simulink model "fangzhen"  (R2018a)
settings: Solver=FixedStepAuto  StartTime=0.0  StopTime=120  FixedStep=0.01  RelTol=1e-3
libraries: simulink x6
(part 2 of 2)

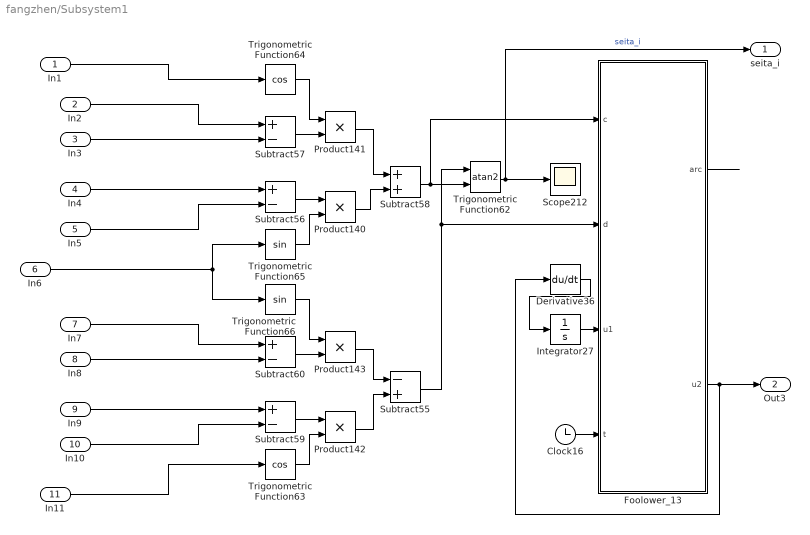
== system fangzhen/Subsystem1 ==
  In1 : Inport
  In2 : Inport  Port=2
  In3 : Inport  Port=3
  In4 : Inport  Port=4
  In5 : Inport  Port=5
  In6 : Inport  Port=6
  In7 : Inport  Port=7
  In8 : Inport  Port=8
  In9 : Inport  Port=9
  In10 : Inport  Port=10
  In11 : Inport  Port=11
  Clock16 : Clock
  Derivative36 : Derivative
  Foolower_13 : MATLAB Function  TreatAsAtomicUnit=on
  Integrator27 : Integrator
  Product{140..143} (4 alike) : Product
  Scope212 : Scope
  Subtract55 : Sum  Inputs=-+
  Subtract{56..57,59..60} (4 alike) : Sum  Inputs=+-
  Subtract58 : Sum
  Trigonometric Function62 : Trigonometry  Operator=atan2
  Trigonometric Function63 : Trigonometry  Operator=cos
  Trigonometric Function64 : Trigonometry  Operator=cos
  Trigonometric Function65 : Trigonometry
  Trigonometric Function66 : Trigonometry
  seita_i : Outport
  Out3 : Outport  Port=2
  wires:
  Foolower_13/2(u2) -> Out3/1, Derivative36/1
  Trigonometric Function64/1 -> Product141/1
  In6/1 -> Trigonometric Function66/1, Trigonometric Function65/1
  Trigonometric Function66/1 -> Product143/1
  Subtract58/1 -> Foolower_13/1(c), Trigonometric Function62/2
  In3/1 -> Subtract57/2
  Product142/1 -> Subtract55/2
  Subtract55/1 -> Trigonometric Function62/1, Foolower_13/2(d)
  Product143/1 -> Subtract55/1
  In10/1 -> Subtract59/2
  Subtract60/1 -> Product143/2
  Derivative36/1 -> Integrator27/1
  In9/1 -> Subtract59/1
  Trigonometric Function63/1 -> Product142/2
  Trigonometric Function62/1 -> seita_i/1, Scope212/1  "seita_i"
  Clock16/1 -> Foolower_13/4(t)
  In1/1 -> Trigonometric Function64/1
  Subtract56/1 -> Product140/1
  Integrator27/1 -> Foolower_13/3(u1)
  In5/1 -> Subtract56/2
  Subtract59/1 -> Product142/1
  Product141/1 -> Subtract58/1
  Foolower_13/1(arc) -> ?
  Product140/1 -> Subtract58/2
  In2/1 -> Subtract57/1
  Trigonometric Function65/1 -> Product140/2
  Subtract57/1 -> Product141/2
  In11/1 -> Trigonometric Function63/1
  In7/1 -> Subtract60/1
  In8/1 -> Subtract60/2
  In4/1 -> Subtract56/1

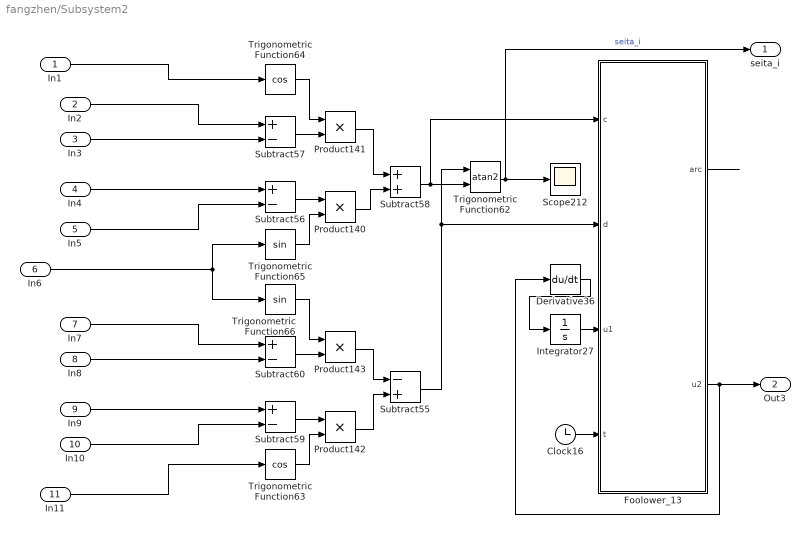
== system fangzhen/Subsystem2 ==
  In1 : Inport
  In2 : Inport  Port=2
  In3 : Inport  Port=3
  In4 : Inport  Port=4
  In5 : Inport  Port=5
  In6 : Inport  Port=6
  In7 : Inport  Port=7
  In8 : Inport  Port=8
  In9 : Inport  Port=9
  In10 : Inport  Port=10
  In11 : Inport  Port=11
  Clock16 : Clock
  Derivative36 : Derivative
  Foolower_13 : MATLAB Function  TreatAsAtomicUnit=on
  Integrator27 : Integrator
  Product{140..143} (4 alike) : Product
  Scope212 : Scope
  Subtract55 : Sum  Inputs=-+
  Subtract{56..57,59..60} (4 alike) : Sum  Inputs=+-
  Subtract58 : Sum
  Trigonometric Function62 : Trigonometry  Operator=atan2
  Trigonometric Function63 : Trigonometry  Operator=cos
  Trigonometric Function64 : Trigonometry  Operator=cos
  Trigonometric Function65 : Trigonometry
  Trigonometric Function66 : Trigonometry
  seita_i : Outport
  Out3 : Outport  Port=2
  wires:
  Foolower_13/2(u2) -> Out3/1, Derivative36/1
  Trigonometric Function64/1 -> Product141/1
  In6/1 -> Trigonometric Function66/1, Trigonometric Function65/1
  Trigonometric Function66/1 -> Product143/1
  Subtract58/1 -> Foolower_13/1(c), Trigonometric Function62/2
  In3/1 -> Subtract57/2
  Product142/1 -> Subtract55/2
  Subtract55/1 -> Trigonometric Function62/1, Foolower_13/2(d)
  Product143/1 -> Subtract55/1
  In10/1 -> Subtract59/2
  Subtract60/1 -> Product143/2
  Derivative36/1 -> Integrator27/1
  In9/1 -> Subtract59/1
  Trigonometric Function63/1 -> Product142/2
  Trigonometric Function62/1 -> seita_i/1, Scope212/1  "seita_i"
  Clock16/1 -> Foolower_13/4(t)
  In1/1 -> Trigonometric Function64/1
  Subtract56/1 -> Product140/1
  Integrator27/1 -> Foolower_13/3(u1)
  In5/1 -> Subtract56/2
  Subtract59/1 -> Product142/1
  Product141/1 -> Subtract58/1
  Foolower_13/1(arc) -> ?
  Product140/1 -> Subtract58/2
  In2/1 -> Subtract57/1
  Trigonometric Function65/1 -> Product140/2
  Subtract57/1 -> Product141/2
  In11/1 -> Trigonometric Function63/1
  In7/1 -> Subtract60/1
  In8/1 -> Subtract60/2
  In4/1 -> Subtract56/1

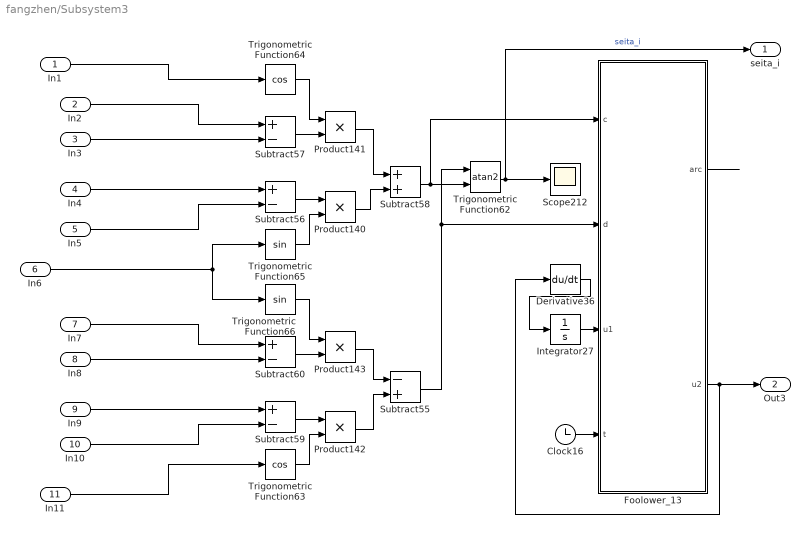
== system fangzhen/Subsystem3 ==
  In1 : Inport
  In2 : Inport  Port=2
  In3 : Inport  Port=3
  In4 : Inport  Port=4
  In5 : Inport  Port=5
  In6 : Inport  Port=6
  In7 : Inport  Port=7
  In8 : Inport  Port=8
  In9 : Inport  Port=9
  In10 : Inport  Port=10
  In11 : Inport  Port=11
  Clock16 : Clock
  Derivative36 : Derivative
  Foolower_13 : MATLAB Function  TreatAsAtomicUnit=on
  Integrator27 : Integrator
  Product{140..143} (4 alike) : Product
  Scope212 : Scope
  Subtract55 : Sum  Inputs=-+
  Subtract{56..57,59..60} (4 alike) : Sum  Inputs=+-
  Subtract58 : Sum
  Trigonometric Function62 : Trigonometry  Operator=atan2
  Trigonometric Function63 : Trigonometry  Operator=cos
  Trigonometric Function64 : Trigonometry  Operator=cos
  Trigonometric Function65 : Trigonometry
  Trigonometric Function66 : Trigonometry
  seita_i : Outport
  Out3 : Outport  Port=2
  wires:
  Foolower_13/2(u2) -> Out3/1, Derivative36/1
  Trigonometric Function64/1 -> Product141/1
  In6/1 -> Trigonometric Function66/1, Trigonometric Function65/1
  Trigonometric Function66/1 -> Product143/1
  Subtract58/1 -> Foolower_13/1(c), Trigonometric Function62/2
  In3/1 -> Subtract57/2
  Product142/1 -> Subtract55/2
  Subtract55/1 -> Trigonometric Function62/1, Foolower_13/2(d)
  Product143/1 -> Subtract55/1
  In10/1 -> Subtract59/2
  Subtract60/1 -> Product143/2
  Derivative36/1 -> Integrator27/1
  In9/1 -> Subtract59/1
  Trigonometric Function63/1 -> Product142/2
  Trigonometric Function62/1 -> seita_i/1, Scope212/1  "seita_i"
  Clock16/1 -> Foolower_13/4(t)
  In1/1 -> Trigonometric Function64/1
  Subtract56/1 -> Product140/1
  Integrator27/1 -> Foolower_13/3(u1)
  In5/1 -> Subtract56/2
  Subtract59/1 -> Product142/1
  Product141/1 -> Subtract58/1
  Foolower_13/1(arc) -> ?
  Product140/1 -> Subtract58/2
  In2/1 -> Subtract57/1
  Trigonometric Function65/1 -> Product140/2
  Subtract57/1 -> Product141/2
  In11/1 -> Trigonometric Function63/1
  In7/1 -> Subtract60/1
  In8/1 -> Subtract60/2
  In4/1 -> Subtract56/1

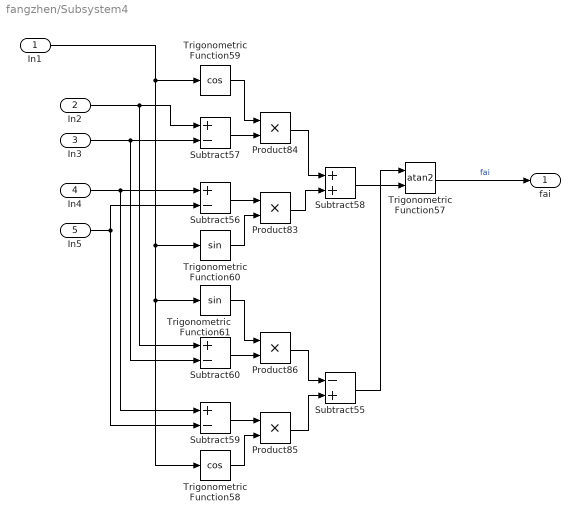
== system fangzhen/Subsystem4 ==
  In1 : Inport
  In2 : Inport  Port=2
  In3 : Inport  Port=3
  In4 : Inport  Port=4
  In5 : Inport  Port=5
  Product{83..86} (4 alike) : Product
  Subtract55 : Sum  Inputs=-+
  Subtract{56..57,59..60} (4 alike) : Sum  Inputs=+-
  Subtract58 : Sum
  Trigonometric Function57 : Trigonometry  Operator=atan2
  Trigonometric Function58 : Trigonometry  Operator=cos
  Trigonometric Function59 : Trigonometry  Operator=cos
  Trigonometric Function60 : Trigonometry
  Trigonometric Function61 : Trigonometry
  fai : Outport
  wires:
  Subtract60/1 -> Product86/2
  Trigonometric Function60/1 -> Product83/2
  Subtract55/1 -> Trigonometric Function57/1
  In1/1 -> Trigonometric Function58/1, Trigonometric Function61/1, Trigonometric Function60/1, Trigonometric Function59/1
  Subtract57/1 -> Product84/2
  Trigonometric Function61/1 -> Product86/1
  Product83/1 -> Subtract58/2
  Product86/1 -> Subtract55/1
  Trigonometric Function59/1 -> Product84/1
  Trigonometric Function58/1 -> Product85/2
  Product84/1 -> Subtract58/1
  In2/1 -> Subtract60/1, Subtract57/1
  Subtract58/1 -> Trigonometric Function57/2
  Subtract56/1 -> Product83/1
  In3/1 -> Subtract60/2, Subtract57/2
  In4/1 -> Subtract59/1, Subtract56/1
  Subtract59/1 -> Product85/1
  Trigonometric Function57/1 -> fai/1  "fai"
  In5/1 -> Subtract59/2, Subtract56/2
  Product85/1 -> Subtract55/2

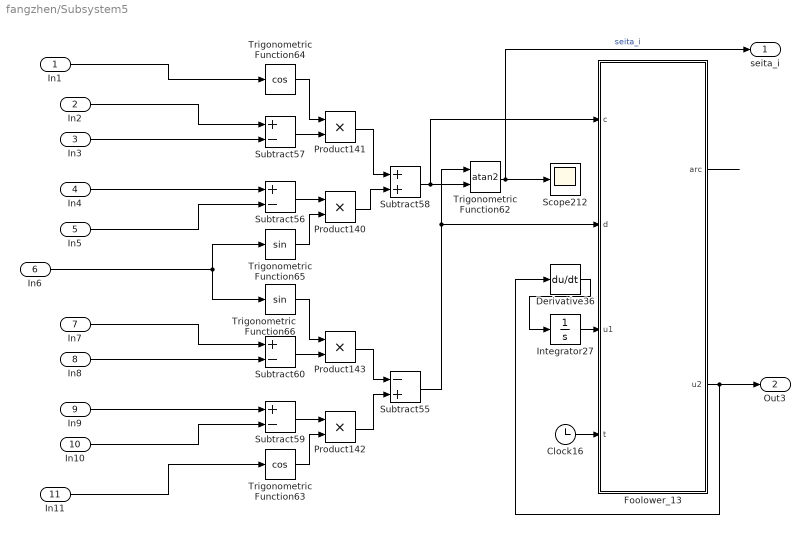
== system fangzhen/Subsystem5 ==
  In1 : Inport
  In2 : Inport  Port=2
  In3 : Inport  Port=3
  In4 : Inport  Port=4
  In5 : Inport  Port=5
  In6 : Inport  Port=6
  In7 : Inport  Port=7
  In8 : Inport  Port=8
  In9 : Inport  Port=9
  In10 : Inport  Port=10
  In11 : Inport  Port=11
  Clock16 : Clock
  Derivative36 : Derivative
  Foolower_13 : MATLAB Function  TreatAsAtomicUnit=on
  Integrator27 : Integrator
  Product{140..143} (4 alike) : Product
  Scope212 : Scope
  Subtract55 : Sum  Inputs=-+
  Subtract{56..57,59..60} (4 alike) : Sum  Inputs=+-
  Subtract58 : Sum
  Trigonometric Function62 : Trigonometry  Operator=atan2
  Trigonometric Function63 : Trigonometry  Operator=cos
  Trigonometric Function64 : Trigonometry  Operator=cos
  Trigonometric Function65 : Trigonometry
  Trigonometric Function66 : Trigonometry
  seita_i : Outport
  Out3 : Outport  Port=2
  wires:
  Foolower_13/2(u2) -> Out3/1, Derivative36/1
  Trigonometric Function64/1 -> Product141/1
  In6/1 -> Trigonometric Function66/1, Trigonometric Function65/1
  Trigonometric Function66/1 -> Product143/1
  Subtract58/1 -> Foolower_13/1(c), Trigonometric Function62/2
  In3/1 -> Subtract57/2
  Product142/1 -> Subtract55/2
  Subtract55/1 -> Trigonometric Function62/1, Foolower_13/2(d)
  Product143/1 -> Subtract55/1
  In10/1 -> Subtract59/2
  Subtract60/1 -> Product143/2
  Derivative36/1 -> Integrator27/1
  In9/1 -> Subtract59/1
  Trigonometric Function63/1 -> Product142/2
  Trigonometric Function62/1 -> seita_i/1, Scope212/1  "seita_i"
  Clock16/1 -> Foolower_13/4(t)
  In1/1 -> Trigonometric Function64/1
  Subtract56/1 -> Product140/1
  Integrator27/1 -> Foolower_13/3(u1)
  In5/1 -> Subtract56/2
  Subtract59/1 -> Product142/1
  Product141/1 -> Subtract58/1
  Foolower_13/1(arc) -> ?
  Product140/1 -> Subtract58/2
  In2/1 -> Subtract57/1
  Trigonometric Function65/1 -> Product140/2
  Subtract57/1 -> Product141/2
  In11/1 -> Trigonometric Function63/1
  In7/1 -> Subtract60/1
  In8/1 -> Subtract60/2
  In4/1 -> Subtract56/1

== matlab function fangzhen/Foolower_2 ==
  data: xl input; ldot output; yl input; xf1head input; yf1head input
function ldot = fcn(xl,yl,xf1head,yf1head)

u=((yl-yf1head)^2+(xl-xf1head)^2)^(1/2);
ldot=u;

== matlab function fangzhen/MATLAB Function1 ==
  data: x0 input; y output; d1 input; jie input; fin input; a output; shangjieyuzhi input; rou input
function [y,a] = fcn(x0,d1,jie,fin,shangjieyuzhi,rou)
if x0>=shangjieyuzhi
    u=d1;a=1;
else
   if x0<shangjieyuzhi&&x0>=shangjieyuzhi-rou
   u=jie;a=2;
    else
     u=fin;a=3;
   end
    
end



y = u;

== matlab function fangzhen/MATLAB Function3 ==
  data: s input; V output; c input; l input; h input; u1 input; u2 input; W output
function [V,W] = fcn(s,c,l,h,u1,u2)


V=-(l+h*c)/(l*c+h)*u1+(h*s*l)/(l*c+h)*u2;

W=-s/(l*c+h)*u1-c*l/(l*c+h)*u2;

== matlab function fangzhen/MATLAB Function ==
  data: x0 input; x0_xia input; thetaid input; theta_shang_xiuzheng input; theta_xia_xiuzheng input; thetaid_0 output; shangjie_yuzhi input; xiajie_yuzhi input; a output
function [thetaid_0,a] = fcn(x0,x0_xia,thetaid,theta_shang_xiuzheng,theta_xia_xiuzheng,shangjie_yuzhi,xiajie_yuzhi)

if x0>=shangjie_yuzhi && x0_xia<=xiajie_yuzhi

  thetaid_0=thetaid;
  a=3;
else
 
  if x0<shangjie_yuzhi && x0_xia<=xiajie_yuzhi
  
   thetaid_0=theta_shang_xiuzheng;
   a=1;
   
else
   thetaid_0=theta_xia_xiuzheng;
   a=2;
   
  end
    
end

== matlab function fangzhen/MATLAB Function15 ==
  data: x0 input; shangjie_yuzhi input; d1u input; d1 output; d1_dotu input; d1_fnu input; d1b input; d1_dot output; d1_fn output; d1_dotb input; d1_fnb input; rou input
function [d1,d1_dot,d1_fn] = fcn(x0,shangjie_yuzhi,d1u,d1_dotu,d1_fnu,d1b,d1_dotb,d1_fnb,rou)
%u输入，b保持
if x0>shangjie_yuzhi

    d1=d1u;
    d1_dot=d1_dotu;
    d1_fn=d1_fnu;
        
else  
    d1=d1b;
    d1_dot=d1_dotb;
    
    if x0>shangjie_yuzhi-rou
     d1_fn=d1_fnu;   
     
    else
     d1_fn=d1_fnb;
    end
    
    
end

== matlab function fangzhen/MATLAB Function2 ==
  data: x0 input; shangjie_yuzhi input; d1u input; d1 output; d1_dotu input; d1_fnu input; d1b input; d1_dot output; d1_fn output; d1_dotb input; d1_fnb input; rou input
function [d1,d1_dot,d1_fn] = fcn(x0,shangjie_yuzhi,d1u,d1_dotu,d1_fnu,d1b,d1_dotb,d1_fnb,rou)
%u输入，b保持
if x0>shangjie_yuzhi

    d1=d1u;
    d1_dot=d1_dotu;
    d1_fn=d1_fnu;
        
else  
    d1=d1b;
    d1_dot=d1_dotb;
    
    if x0>shangjie_yuzhi-rou
     d1_fn=d1_fnu;   
     
    else
     d1_fn=d1_fnb;
    end
    
    
end

== matlab function fangzhen/Subsystem1/Foolower_13 ==
  data: c input; arc output; d input; u1 input; t input; u2 output
function [arc,u2] = fcn(c,d,u1,t)

u=atan2(d,c);
u2=u;
a=u1/pi/2+1;
b=ceil(a+0.2);
% if u<u1
%     u2=2*pi+u;
% end


% if u<0
%     u2=2*pi+u;
% end


arc=u2;

% if u<=0&&b==2
%     u2=4*pi+u;
% end

== matlab function fangzhen/Foolower_1 ==
  data: xl input; ldot output; yl input; xf1head input; yf1head input
function ldot = fcn(xl,yl,xf1head,yf1head)

u=((yl-yf1head)^2+(xl-xf1head)^2)^(1/2);
ldot=u;

== matlab function fangzhen/MATLAB Function10 ==
  data: s input; V output; c input; l input; h input; u1 input; u2 input; W output
function [V,W] = fcn(s,c,l,h,u1,u2)


V=-(l+h*c)/(l*c+h)*u1+(h*s*l)/(l*c+h)*u2;

W=-s/(l*c+h)*u1-c*l/(l*c+h)*u2;

== matlab function fangzhen/Foolower_3 ==
  data: xl input; ldot output; yl input; xf1head input; yf1head input
function ldot = fcn(xl,yl,xf1head,yf1head)

u=((yl-yf1head)^2+(xl-xf1head)^2)^(1/2);
ldot=u;

== matlab function fangzhen/MATLAB Function13 ==
  data: shang_ output; xia_ output; x0 input; x0_xia input; shang input; xia input; shangjie_yuzhi input; xiajie_yuzhi input; a output; shangjie input; xiajie input; shangjie_1 input; xiajie_1 input; shangjie_ output; xiajie_ output
function [shang_,xia_,a,shangjie_,xiajie_] = fcn(x0,x0_xia,shang,xia,shangjie_yuzhi,xiajie_yuzhi,shangjie,xiajie,shangjie_1,xiajie_1)

if x0>=shangjie_yuzhi && x0_xia<=xiajie_yuzhi
 shang_=x0;
 xia_=x0_xia;
 
  shangjie_=shangjie;
  xiajie_=xiajie;
  
  a=3;
else
    
    if x0<shangjie_yuzhi %&& x0_xia<=xiajie_yuzhi
   shang_=shang;
 xia_=xia;
 
    shangjie_=shangjie_1;
  xiajie_=xiajie;
  
   a=1;
   
else
     shang_=shang;
 xia_=xia;
 
  shangjie_=shangjie;
  xiajie_=xiajie_1;
  
   a=2;
   
    end
    
end

== matlab function fangzhen/MATLAB Function7 ==
  data: x0 input; x0_xia input; thetaid input; theta_shang_xiuzheng input; theta_xia_xiuzheng input; thetaid_0 output; shangjie_yuzhi input; xiajie_yuzhi input; a output
function [thetaid_0,a] = fcn(x0,x0_xia,thetaid,theta_shang_xiuzheng,theta_xia_xiuzheng,shangjie_yuzhi,xiajie_yuzhi)

if x0>=shangjie_yuzhi && x0_xia<=xiajie_yuzhi

  thetaid_0=thetaid;
  a=3;
else
 
  if x0<shangjie_yuzhi && x0_xia<=xiajie_yuzhi
  
   thetaid_0=theta_shang_xiuzheng;
   a=1;
   
else
   thetaid_0=theta_xia_xiuzheng;
   a=2;
   
  end
    
end

== matlab function fangzhen/MATLAB Function14 ==
  data: s input; V output; c input; l input; h input; u1 input; u2 input; W output
function [V,W] = fcn(s,c,l,h,u1,u2)


V=-(l+h*c)/(l*c+h)*u1+(h*s*l)/(l*c+h)*u2;

W=-s/(l*c+h)*u1-c*l/(l*c+h)*u2;

== matlab function fangzhen/Subsystem2/Foolower_13 ==
  data: c input; arc output; d input; u1 input; t input; u2 output
function [arc,u2] = fcn(c,d,u1,t)

u=atan2(d,c);
u2=u;
a=u1/pi/2+1;
b=ceil(a+0.2);
% if u<u1
%     u2=2*pi+u;
% end


% if u<0
%     u2=2*pi+u;
% end


arc=u2;

% if u<=0&&b==2
%     u2=4*pi+u;
% end

== matlab function fangzhen/MATLAB Function16 ==
  data: x0 input; y output; d1 input; jie input; fin input; a output; xiajieyuzhi input; rou input
function [y,a] = fcn(x0,d1,jie,fin,xiajieyuzhi,rou)
if x0<=xiajieyuzhi
    u=d1;a=1;
else
    
   if x0>xiajieyuzhi&&x0<=xiajieyuzhi+rou
   u=jie;a=2;
    else
     u=fin;a=3;
   end
    
end



y = u;

== matlab function fangzhen/MATLAB Function17 ==
  data: x0 input; xiajie_yuzhi input; d1u input; d1 output; d1_dotu input; d1_fnu input; d1b input; d1_dot output; d1_fn output; d1_dotb input; d1_fnb input; rou input
function [d1,d1_dot,d1_fn] = fcn(x0,xiajie_yuzhi,d1u,d1_dotu,d1_fnu,d1b,d1_dotb,d1_fnb,rou)
%u输入，b保持
if x0<xiajie_yuzhi

    d1=d1u;
    d1_dot=d1_dotu;
    d1_fn=d1_fnu;
        
else  
    
    d1=d1b;
    d1_dot=d1_dotb;
    
    if x0<xiajie_yuzhi+rou
     d1_fn=d1_fnu;   
     
    else
     d1_fn=d1_fnb;
    end
    
    
end

== matlab function fangzhen/MATLAB Function4 ==
  data: x0 input; y output; d1 input; jie input; fin input; a output; shangjie input; rou input
function [y,a] = fcn(x0,d1,jie,fin,shangjie,rou)
if x0>=shangjie
    u=d1;a=1;
else
   if x0<shangjie&&x0>=shangjie-rou
   u=jie;a=2;
    else
     u=fin;a=3;
   end
    
end



y = u;

== matlab function fangzhen/MATLAB Function20 ==
  data: d1 input; d_ input; d output; shangjie input; xiajie input; a output
function [d,a]  = fcn(d1,d_,shangjie,xiajie)
%此处的下界和上界和拼音无关
 if d1>=xiajie&&d1<=shangjie;
  d=d1;
  a=3;
else
    
    if d1>shangjie
   d=shangjie;
  
   a=1;
   
    else
    
    d=xiajie;
  
   a=2;
   
    end
    
end

== matlab function fangzhen/MATLAB Function22 ==
  data: VL input; y output; Vi input; fai input; pesai input; oumiga_i input; oumiga_L input; h input; L input
function y = fcn(VL,Vi,fai,pesai,oumiga_i,oumiga_L,h,L)

e_pesai_dot = -oumiga_i+(  -VL*sin(fai)+Vi*sin(pesai)-h*oumiga_i*cos(pesai)+h*oumiga_L*cos(fai)    )/L;




y = e_pesai_dot;

== matlab function fangzhen/MATLAB Function23 ==
  data: VL input; y output; Vi input; fai input; pesai input; oumiga_i input; oumiga_L input; h input
function y = fcn(VL,Vi,fai,pesai,oumiga_i,oumiga_L,h)

el_dot=VL*cos(fai)-Vi*cos(pesai)-h*sin(pesai)*oumiga_i+h*oumiga_L*sin(fai);




y = el_dot;

== matlab function fangzhen/MATLAB Function8 ==
  data: d1 input; d output; shangjie input; xiajie input; a output
function [d,a]  = fcn(d1,shangjie,xiajie)
%此处的下界和上界和拼音无关
 if d1>=xiajie&&d1<=shangjie
  d=d1;
  a=3;
else
    
    if d1>shangjie
        
   d=shangjie;
  
   a=1;
   
    else
    
    d=xiajie;
  
   a=2;
   
    end
    
end

== matlab function fangzhen/Subsystem3/Foolower_13 ==
  data: c input; arc output; d input; u1 input; t input; u2 output
function [arc,u2] = fcn(c,d,u1,t)

u=atan2(d,c);
u2=u;
a=u1/pi/2+1;
b=ceil(a+0.2);
% if u<u1
%     u2=2*pi+u;
% end


% if u<0
%     u2=2*pi+u;
% end


arc=u2;

% if u<=0&&b==2
%     u2=4*pi+u;
% end

== matlab function fangzhen/MATLAB Function25 ==
  data: VL input; y output; Vi input; fai input; pesai input; oumiga_i input; oumiga_L input; h input; L input
function y = fcn(VL,Vi,fai,pesai,oumiga_i,oumiga_L,h,L)

e_pesai_dot = -oumiga_i+(  -VL*sin(fai)+Vi*sin(pesai)-h*oumiga_i*cos(pesai)+h*oumiga_L*cos(fai)    )/L;




y = e_pesai_dot;

== matlab function fangzhen/MATLAB Function26 ==
  data: VL input; y output; Vi input; fai input; pesai input; oumiga_i input; oumiga_L input; h input
function y = fcn(VL,Vi,fai,pesai,oumiga_i,oumiga_L,h)

el_dot=VL*cos(fai)-Vi*cos(pesai)-h*sin(pesai)*oumiga_i+h*oumiga_L*sin(fai);




y = el_dot;

== matlab function fangzhen/MATLAB Function27 ==
  data: u input; y output
function y = fcn(u)
 
xa0=x0.signals.values;
xa1=x1.signals.values;
xa2=x2.signals.values;
xa3=x3.signals.values;
xb0=y0.signals.values;
xb1=y1.signals.values;
xb2=y2.signals.values;
xb3=y3.signals.values;
plot(xa0,xb0,xa1,xb1,xa2,xb2,xa3,xb3)

== matlab function fangzhen/MATLAB Function29 ==
  data: VL input; y output; Vi input; fai input; pesai input; oumiga_i input; oumiga_L input; h input; L input
function y = fcn(VL,Vi,fai,pesai,oumiga_i,oumiga_L,h,L)

e_pesai_dot = -oumiga_i+(  -VL*sin(fai)+Vi*sin(pesai)-h*oumiga_i*cos(pesai)+h*oumiga_L*cos(fai)    )/L;




y = e_pesai_dot;

== matlab function fangzhen/MATLAB Function30 ==
  data: VL input; y output; Vi input; fai input; pesai input; oumiga_i input; oumiga_L input; h input
function y = fcn(VL,Vi,fai,pesai,oumiga_i,oumiga_L,h)

el_dot=VL*cos(fai)-Vi*cos(pesai)-h*sin(pesai)*oumiga_i+h*oumiga_L*sin(fai);




y = el_dot;

== matlab function fangzhen/MATLAB Function32 ==
  data: zhouju input; t1 output; r input; m input; Iz input; v_dot input; oumiga_dot input; t2 output
function [t1,t2] = fcn(zhouju,r,m,Iz,v_dot,oumiga_dot)

t1=v_dot*m*r/2-oumiga_dot*Iz*r/2/zhouju;
t2=v_dot*m*r/2+oumiga_dot*Iz*r/2/zhouju;

== matlab function fangzhen/MATLAB Function36 ==
  data: x0 input; shangjie_yuzhi input; d1u input; d1 output; d1_dotu input; d1_fnu input; d1b input; d1_dot output; d1_fn output; d1_dotb input; d1_fnb input; a output; rou input
function [d1,d1_dot,d1_fn,a] = fcn(x0,shangjie_yuzhi,d1u,d1_dotu,d1_fnu,d1b,d1_dotb,d1_fnb,rou)
%u输入，b保持
if x0<=-shangjie_yuzhi

    d1=d1u;
    d1_dot=d1_dotu;
    d1_fn=d1_fnu;
        a=1;
else  
    d1=d1b;
    d1_dot=d1_dotb;
    
    if x0>-shangjie_yuzhi&&x0<-shangjie_yuzhi+rou
     d1_fn=d1_fnu;   
     a=2;
    else
     d1_fn=d1_fnb;
     a=3;
    end
    
    
end

== matlab function fangzhen/MATLAB Function37 ==
  data: x0 input; y output; d1 input; jie input; fin input; a output; xiajie_yuzhi input; rou input
function [y,a] = fcn(x0,d1,jie,fin,xiajie_yuzhi,rou)
if x0>=-xiajie_yuzhi%-0.1
    u=d1;a=1;
else
    
   if x0<-xiajie_yuzhi&&x0>=-xiajie_yuzhi+rou
       %-0.1&&x0>=-0.15
   u=jie;a=2;
    else
     u=fin;a=3;
   end
    
end



y = u;

== matlab function fangzhen/MATLAB Function38 ==
  data: x0 input; xiajie_yuzhi input; d1u input; d1 output; d1_dotu input; d1_fnu input; d1b input; d1_dot output; d1_fn output; d1_dotb input; d1_fnb input; a output; rou input
function [d1,d1_dot,d1_fn,a] = fcn(x0,xiajie_yuzhi,d1u,d1_dotu,d1_fnu,d1b,d1_dotb,d1_fnb,rou)
%u输入，b保持
if x0>=-xiajie_yuzhi

    d1=d1u;
    d1_dot=d1_dotu;
    d1_fn=d1_fnu;
       a=1 ;
else  

    d1=d1b;
    d1_dot=d1_dotb;
    
    if x0<-xiajie_yuzhi&&x0>=-xiajie_yuzhi-rou
       
     d1_fn=d1_fnu;   
         a=2;
    else
     d1_fn=d1_fnb;
     a=3;
    end
    
    
end

== matlab function fangzhen/MATLAB Function39 ==
  data: x0 input; y output; d1 input; jie input; fin input; a output; shangjie_yuzhi input; rou input
function [y,a] = fcn(x0,d1,jie,fin,shangjie_yuzhi,rou)
if x0<=-shangjie_yuzhi
    u=d1;a=1;
else
    
   if x0>-shangjie_yuzhi&&x0<=-shangjie_yuzhi+rou%x0<0.1&&x0>=0.05
       
   u=jie;a=2;
    else
     u=fin;a=3;
   end
    
end



y = u;

% function [y,a] = fcn(x0,d1,jie,fin)
% if x0>=0.1
%     u=d1;a=1;
% else
%    if x0<0.1&&x0>=0.05
%    u=jie;a=2;
%     else
%      u=fin;a=3;
%    end
%     
% end
% 
% 
% 
% y = u;

== matlab function fangzhen/Subsystem5/Foolower_13 ==
  data: c input; arc output; d input; u1 input; t input; u2 output
function [arc,u2] = fcn(c,d,u1,t)

u=atan2(d,c);
u2=u;
a=u1/pi/2+1;
b=ceil(a+0.2);
% if u<u1
%     u2=2*pi+u;
% end


% if u<0
%     u2=2*pi+u;
% end


arc=u2;

% if u<=0&&b==2
%     u2=4*pi+u;
% end

== matlab function fangzhen/MATLAB Function47 ==
  data: zhouju input; t1 output; r input; m input; Iz input; v_dot input; oumiga_dot input; t2 output
function [t1,t2] = fcn(zhouju,r,m,Iz,v_dot,oumiga_dot)

t1=v_dot*m*r/2-oumiga_dot*Iz*r/2/zhouju;
t2=v_dot*m*r/2+oumiga_dot*Iz*r/2/zhouju;

== matlab function fangzhen/MATLAB Function48 ==
  data: x0 input; y output; d1 input; jie input; fin input; a output; xiajieyuzhi input; rou input
function [y,a] = fcn(x0,d1,jie,fin,xiajieyuzhi,rou)
if x0<=xiajieyuzhi
    u=d1;a=1;
else
    
   if x0>xiajieyuzhi&&x0<=xiajieyuzhi-rou
   u=jie;a=2;
    else
     u=fin;a=3;
   end
    
end



y = u;

== matlab function fangzhen/MATLAB Function49 ==
  data: x0 input; xiajie_yuzhi input; d1u input; d1 output; d1_dotu input; d1_fnu input; d1b input; d1_dot output; d1_fn output; d1_dotb input; d1_fnb input; rou input
function [d1,d1_dot,d1_fn] = fcn(x0,xiajie_yuzhi,d1u,d1_dotu,d1_fnu,d1b,d1_dotb,d1_fnb,rou)
%u输入，b保持
if x0<xiajie_yuzhi

    d1=d1u;
    d1_dot=d1_dotu;
    d1_fn=d1_fnu;
        
else  
    
    d1=d1b;
    d1_dot=d1_dotb;
    
    if x0<xiajie_yuzhi+rou
     d1_fn=d1_fnu;   
     
    else
     d1_fn=d1_fnb;
    end
    
    
end

== matlab function fangzhen/Foolower_4 ==
  data: x2 input; arc output; y2 input; x1 input; y1 input; u1 input; u2 output; c1 input; s1 input
function [arc,u2] = fcn(x2,y2,x1,y1,u1,c1,s1)
%注意：求解（3,5）的坐标需要输入（5,3）
% 注意：x2-x1是正的y2-y1是负的
x=(-c1*(x2-x1)+s1*(y1-y2));
y=(s1*(x2-x1)+c1*(y1-y2));
u=atan2(x,y);

u2=u;
a=u1/pi/2+1;
b=ceil(a+0.2);

% if u>u1
%     u2=2*pi+u;
% end
% if u<0
%     u2=2*pi+u;
% end



arc=u2;

== matlab function fangzhen/MATLAB Function50 ==
  data: x input; y output; y input
function y = fcn(x,y)
u=atan2(x,y);
y = u;

== matlab function fangzhen/Foolower_5 ==
  data: xl input; ldot output; yl input; xf1head input; yf1head input
function ldot = fcn(xl,yl,xf1head,yf1head)

u=((yl-yf1head)^2+(xl-xf1head)^2)^(1/2);
ldot=u;

== matlab function fangzhen/MATLAB Function52 ==
  data: zhouju input; t1 output; r input; m input; Iz input; v_dot input; oumiga_dot input; t2 output
function [t1,t2] = fcn(zhouju,r,m,Iz,v_dot,oumiga_dot)

t1=v_dot*m*r/2-oumiga_dot*Iz*r/2/zhouju;
t2=v_dot*m*r/2+oumiga_dot*Iz*r/2/zhouju;

== matlab function fangzhen/MATLAB 需要跑30s6 ==
  data: ks input; y output; t input; a output; s input
function [y,a] = fcn(ks,t,s)
    b=0;
%使用积分得到目标曲线的转角，之后设计原函数和自变量
if t<=10
    u=0;
    a=1;

elseif t>10&&t<=60
      u=pi*(t-10)/1400;
      a=2;
elseif t>60&&t<=110
      u=pi*(110-t)/1400;
      a=3;
   

 else
    u=0;
    a=8;
      
      
end
y = u;


% function [y,a] = fcn(ks,t)
%     b=0;
% if t<=10
%     u=0;
%     a=1;
% 
% elseif t>10&&t<=260
%      u=ks*(t-10);
%      a=2;
% elseif t>260&&t<=300
%       u=ks*250;
%       a=3;
% elseif t>300&&t<=350
%       u=ks*250*(350-t)/50;
%       a=4;
% elseif t>350+b&&t<=400
%     u=ks*250*(350-t)/50;
%       a=5;
% elseif t>400&&t<=440
%       u=-ks*250;
%       a=6;
% elseif t>440+b&&t<=690+b
%       u=-ks*(690-t);
%       a=7;
% else
%     u=0;
%     a=8;
%       
%       
% end
% y = u;
%
